simulink model "GbxFr"  (R2020b)
settings: configuration reference "gen_config" (kept outside this file)
undefined symbols (not defined in the file): GbxFr_tqClutchMax_C
settings Model: DataDictionary=Hybrid_vehicle.sldd  SimulationMode=accelerator  Creator=Georg  LastModifiedBy=jy
settings ConfigSetRef: SourceName=gen_config

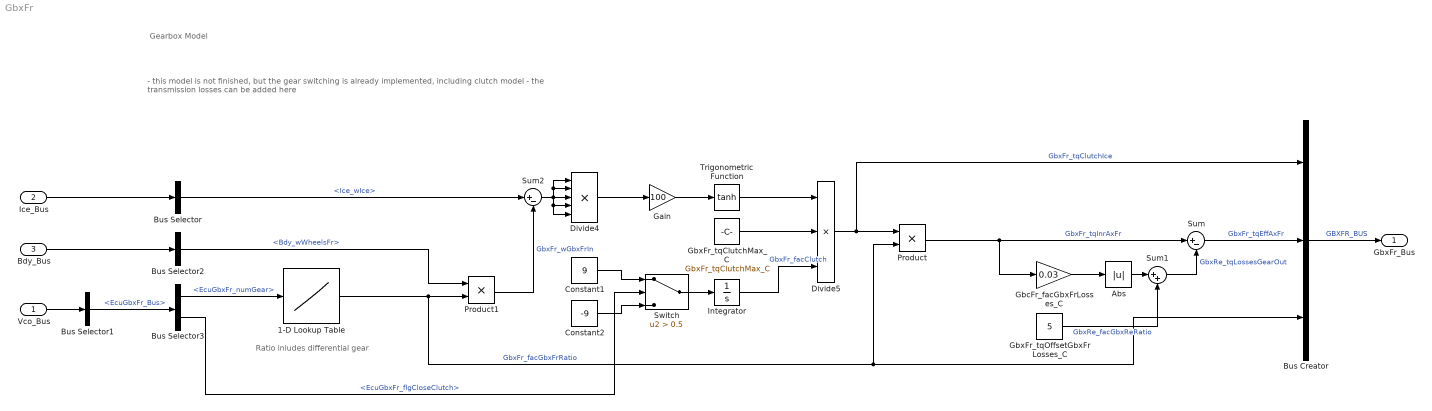
== system GbxFr ==
  note: Ratio inludes differential gear
  note: Gearbox Model
  note: - this model is not finished, but the gear switching is already implemented, including clutch model
      | - the transmission losses can be added here
  Vco_Bus : Inport  OutDataTypeStr=Bus: VCO_BUS
  Ice_Bus : Inport  Port=2  OutDataTypeStr=Bus: ICE_BUS
  Bdy_Bus : Inport  Port=3  OutDataTypeStr=Bus: BDY_BUS
  1-D Lookup Table : Lookup_n-D  NumberOfTableDimensions=1  BreakpointsForDimension1=[1 2 3 4 5]  Table="[12.144\t7.155392\t4.812336\t3.788192\t3.080896]"  InterpMethod=Nearest  InternalRulePriority=Speed  RndMeth=Simplest  InputSameDT=on
  Abs : Abs
  Bus Creator : BusCreator  Inputs=3  OutDataTypeStr=Bus: GBXFR_BUS
  Bus Selector : BusSelector  OutputSignals=Ice_wIce
  Bus Selector1 : BusSelector  OutputSignals=EcuGbxFr_Bus
  Bus Selector2 : BusSelector  OutputSignals=Bdy_wWheelsFr
  Bus Selector3 : BusSelector  OutputSignals=EcuGbxFr_numGear,EcuGbxFr_flgCloseClutch
  Constant1 : Constant  Value=9
  Constant2 : Constant  Value=-9
  Divide4 : Product  Inputs=*****
  Divide5 : Product  Inputs=***
  Gain : Gain  Gain=100
  GbcFr_facGbxFrLosses_C : Gain  Gain=0.03
  GbxFr_tqClutchMax_C : Constant  Value=GbxFr_tqClutchMax_C
  GbxFr_tqOffsetGbxFrLosses_C : Constant  Value=5
  Integrator : Integrator  LimitOutput=on  UpperSaturationLimit=1  LowerSaturationLimit=0
  Product : Product
  Product1 : Product
  Sum : Sum  Inputs=|+-
  Sum1 : Sum  Inputs=|++
  Sum2 : Sum  Inputs=|+-
  Switch : Switch  Criteria=u2 > Threshold  Threshold=0.5
  Trigonometric Function : Trigonometry  Operator=tanh
  GbxFr_Bus : Outport  OutDataTypeStr=Bus: GBXFR_BUS  VectorParamsAs1DForOutWhenUnconnected=off
  wires:
  Trigonometric Function/1 -> Divide5/1
  GbcFr_facGbxFrLosses_C/1 -> Abs/1
  Sum1/1 -> Sum/2  "GbxRe_tqLossesGearOut"
  Abs/1 -> Sum1/1
  Integrator/1 -> Divide5/3  "GbxFr_facClutch"
  Bus Selector1/1 -> Bus Selector3/1  "<EcuGbxFr_Bus>"
  Bus Selector3/1 -> 1-D Lookup Table/1  "<EcuGbxFr_numGear>"
  Product/1 -> GbcFr_facGbxFrLosses_C/1, Sum/1  "GbxFr_tqInrAxFr"
  Sum2/1 -> Divide4/5, Divide4/4, Divide4/1, Divide4/2, Divide4/3
  GbxFr_tqOffsetGbxFrLosses_C/1 -> Sum1/2  "GbxRe_facGbxReRatio"
  Constant1/1 -> Switch/1
  GbxFr_tqClutchMax_C/1 -> Divide5/2
  Divide4/1 -> Gain/1
  Sum/1 -> Bus Creator/2  "GbxFr_tqEffAxFr"
  Bus Creator/1 -> GbxFr_Bus/1  "GBXFR_BUS"
  Bus Selector2/1 -> Product1/1  "<Bdy_wWheelsFr>"
  Divide5/1 -> Product/1, Bus Creator/1  "GbxFr_tqClutchIce"
  Product1/1 -> Sum2/2  "GbxFr_wGbxFrIn"
  Gain/1 -> Trigonometric Function/1
  Switch/1 -> Integrator/1
  Constant2/1 -> Switch/3
  Vco_Bus/1 -> Bus Selector1/1
  Ice_Bus/1 -> Bus Selector/1
  Bus Selector/1 -> Sum2/1  "<Ice_wIce>"
  Bus Selector3/2 -> Switch/2  "<EcuGbxFr_flgCloseClutch>"
  Bdy_Bus/1 -> Bus Selector2/1
  1-D Lookup Table/1 -> Product1/2, Product/2, Bus Creator/3  "GbxFr_facGbxFrRatio"
